simulink model "New_Control_Law_I_StandAlone"  (R2014a)
settings: configuration reference "AR_Drone_ConfigSet_NOEXT" (kept outside this file)
values from neighbouring files (symbols this model uses):
  Accel_Calib_Gain = Simulink.Parameter    [AR_DRONE_SCRIPT.m]
  Accel_Calib_Offset = Simulink.Parameter    [AR_DRONE_SCRIPT.m]
undefined symbols (not defined in the file or in its folder): Mag_Calib_Gain_Vector, Mag_Calib_Offset_Vector, Navigation, Navigation_KF_Lib, sigbuilder_block
libraries: simulink x14, vrlib x6, AR_Drone_2_Library x4, aerolibtransform2 x4, dspnetwork x4, aerolibutil x2
(part 1 of 3)
settings Model: ExtModeTrigDuration=48000  Creator=nraman  LastModifiedBy=darenlee

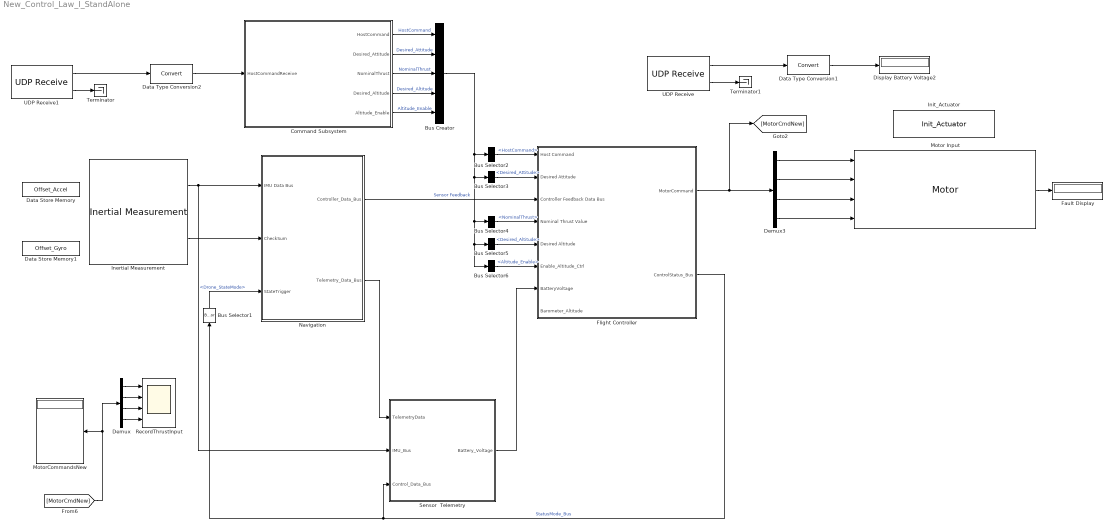
== system New_Control_Law_I_StandAlone ==
  Bus Creator : BusCreator  Inputs=5
  Bus Selector1 : BusSelector  OutputSignals=Drone_StateMode
  Bus Selector2 : BusSelector  OutputSignals=HostCommand
  Bus Selector3 : BusSelector  OutputSignals=Desired_Attitude
  Bus Selector4 : BusSelector  OutputSignals=NominalThrust
  Bus Selector5 : BusSelector  OutputSignals=Desired_Altitude
  Bus Selector6 : BusSelector  OutputSignals=Altitude_Enable
  Command Subsystem : Subsystem
  Data Store Memory : DataStoreMemory  DataStoreName=Offset_Accel  ReadBeforeWriteMsg=warning  WriteAfterWriteMsg=warning  WriteAfterReadMsg=warning  InitialValue=[0 0]  OutDataTypeStr=double
  Data Store Memory1 : DataStoreMemory  DataStoreName=Offset_Gyro  ReadBeforeWriteMsg=warning  WriteAfterWriteMsg=warning  WriteAfterReadMsg=warning  InitialValue=[0 0 0]  OutDataTypeStr=double
  Data Type Conversion1 : DataTypeConversion
  Data Type Conversion2 : DataTypeConversion
  Demux : Demux
  Demux3 : Demux
  Display Battery Voltage2 : Display
  Fault Display : Display
  Flight Controller : Subsystem
  Inertial Measurement : AR_Drone_2_Library/Inertial Measurement  Ts=1/400
  Init_Actuator : AR_Drone_2_Library/Init_Actuator  ShowSpec=on
  Motor Input : AR_Drone_2_Library/Motor
  MotorCommandsNew : Display
  Navigation : Subsystem  AncestorBlock=Navigation_KF_Lib/Navigation
      mask DialogControl DescTextVar Prompt: Kalman Filter Navigation Implementation
  RecordThrustInput : Scope  NumInputPorts=4
      settings: TimeRange=44.32823813354787  YMin=20~20~-5~-5  YMax=85~90~5~5  SaveName=Control_Input
  Sensor  Telemetry : Subsystem
  Terminator : Terminator
  Terminator1 : Terminator
  UDP Receive : dspnetwork/UDP Receive  localURL='0.0.0.0'  localPort=6000  remoteURL='192.168.1.2'  remotePort=-1  recvBufferSize=8192  dims=1  signalDatatype=int8  isVarSize=off  showBlockingTime=on  blockingTime=0  sampletime=1/400  blockPlatform=LINUX
  UDP Receive1 : dspnetwork/UDP Receive  localURL='0.0.0.0'  localPort=6000  remoteURL='192.168.1.2'  remotePort=-1  recvBufferSize=8192  dims=1  signalDatatype=int8  isVarSize=off  showBlockingTime=on  blockingTime=0  sampletime=1/400  blockPlatform=LINUX
  wires:
  Motor Input/1 -> Fault Display/1
  Demux3/1 -> Motor Input/1
  Demux3/2 -> Motor Input/2
  Demux3/3 -> Motor Input/3
  Demux3/4 -> Motor Input/4
  Inertial Measurement/1 -> Sensor  Telemetry/2(IMU_Bus), Navigation/1(IMU Data Bus)
  Inertial Measurement/2 -> Navigation/2(CheckSum)
  Bus Creator/1 -> Bus Selector2/1, Bus Selector3/1, Bus Selector4/1, Bus Selector6/1, Bus Selector5/1
  Bus Selector4/1 -> Flight Controller/4(Nominal Thrust Value)  "<NominalThrust>"
  Bus Selector5/1 -> Flight Controller/5(Desired Altitude)  "<Desired_Altitude>"
  Bus Selector6/1 -> Flight Controller/6(Enable_Altitude_Ctrl)  "<Altitude_Enable>"
  Flight Controller/1(MotorCommand) -> [MotorCmdNew], Demux3/1
  Flight Controller/2(ControlStatus_Bus) -> Sensor  Telemetry/3(Control_Data_Bus), Bus Selector1/1  "StatusMode_Bus"
  Bus Selector1/1 -> Navigation/3(StateTrigger)  "<Drone_StateMode>"
  [MotorCmdNew] -> MotorCommandsNew/1, Demux/1
  Demux/1 -> RecordThrustInput/1
  Demux/2 -> RecordThrustInput/2
  Demux/3 -> RecordThrustInput/3
  Demux/4 -> RecordThrustInput/4
  Command Subsystem/1(HostCommand) -> Bus Creator/1  "HostCommand"
  Command Subsystem/2(Desired_Attitude) -> Bus Creator/2  "Desired_Attitude"
  Command Subsystem/3(NominalThrust) -> Bus Creator/3  "NominalThrust"
  Command Subsystem/4(Desired_Altitude) -> Bus Creator/4  "Desired_Altitude"
  Command Subsystem/5(Altitude_Enable) -> Bus Creator/5  "Altitude_Enable"
  Bus Selector2/1 -> Flight Controller/1(Host Command)  "<HostCommand>"
  Bus Selector3/1 -> Flight Controller/2(Desired Attitude)  "<Desired_Attitude>"
  Navigation/1(Controller_Data_Bus) -> Flight Controller/3(Controller Feedback Data Bus)  "Sensor Feedback"
  Navigation/2(Telemetry_Data_Bus) -> Sensor  Telemetry/1(TelemetryData)
  UDP Receive/1 -> Data Type Conversion1/1
  Data Type Conversion1/1 -> Display Battery Voltage2/1
  Sensor  Telemetry/1(Battery_Voltage) -> Flight Controller/7(BatteryVoltage)
  UDP Receive1/1 -> Data Type Conversion2/1
  Data Type Conversion2/1 -> Command Subsystem/1(HostCommandReceive)
  UDP Receive1/2 -> Terminator/1
  UDP Receive/2 -> Terminator1/1

== system New_Control_Law_I_StandAlone/Command Subsystem ==
  HostCommandReceive : Inport
  Altitude_OFF : Constant  Value=0
  Altitude_ON : Constant
  Data Type Conversion5 : DataTypeConversion
  Desired Attitude : Subsystem
  Desired Euler Angle Attitude1 : Constant  Value=120
  Desired Euler Angle Attitude2 : Constant  Value=50
  Enable/Disable Altitude : ManualSwitch
  Go High : Constant
  Go Low : Constant  Value=0
  Height Control : ManualSwitch
  Nominal Thrust1 : Constant  Value=55
  Switch1 : Switch  Criteria=u2 > Threshold
  HostCommand : Outport
  Desired_Attitude : Outport  Port=2
  NominalThrust : Outport  Port=3
  Desired_Altitude : Outport  Port=4
  Altitude_Enable : Outport  Port=5
  wires:
  Desired Euler Angle Attitude2/1 -> Switch1/3
  Height Control/1 -> Switch1/2
  Desired Euler Angle Attitude1/1 -> Switch1/1
  Go High/1 -> Height Control/1
  Go Low/1 -> Height Control/2
  Altitude_OFF/1 -> Enable/Disable Altitude/2
  Altitude_ON/1 -> Enable/Disable Altitude/1
  Switch1/1 -> Desired_Altitude/1
  Enable/Disable Altitude/1 -> Altitude_Enable/1
  Nominal Thrust1/1 -> NominalThrust/1
  Desired Attitude/1(Ref_Attitude) -> Data Type Conversion5/1
  Data Type Conversion5/1 -> Desired_Attitude/1
  HostCommandReceive/1 -> HostCommand/1

== system New_Control_Law_I_StandAlone/Flight Controller ==
  Host Command : Inport
  Desired Attitude : Inport  Port=2
  Controller Feedback Data Bus : Inport  Port=3
  Nominal Thrust Value : Inport  Port=4
  Desired Altitude : Inport  Port=5
  Enable_Altitude_Ctrl : Inport  Port=6
  BatteryVoltage : Inport  Port=7
  Barometer_Altitude : Inport  Port=8
  Bus Creator : BusCreator  Inputs=5
  Bus Selector : BusSelector  OutputSignals=UltraSound,EulerAngles,ProcessedGyro,AccelNorm
  FilterBattVoltage : DiscreteTransferFcn  Numerator=[ 0.07226]  Denominator=[1 -0.9277]  SampleTime=1/400
  Selector : Selector  InputPortWidth=3  Indices=[3]
  Supervisory Flight Controller : Stateflow chart  TreatAsAtomicUnit=on
  Terminator : Terminator
  MotorCommand : Outport
  ControlStatus_Bus : Outport  Port=2
  wires:
  Supervisory Flight Controller/1(MotorCmd) -> Bus Creator/1, MotorCommand/1
  Desired Attitude/1 -> Supervisory Flight Controller/2(Desired_Attitude_deg)
  Desired Altitude/1 -> Supervisory Flight Controller/9(Desired_Altitude)
  Supervisory Flight Controller/2(" Drone_StateMode") -> Bus Creator/2
  Host Command/1 -> Supervisory Flight Controller/1(hostCmd)
  Bus Selector/1 -> Supervisory Flight Controller/3(UltraSound_Feedback)  "<UltraSound>"
  Nominal Thrust Value/1 -> Supervisory Flight Controller/7(NominalThrust)
  Controller Feedback Data Bus/1 -> Bus Selector/1
  Enable_Altitude_Ctrl/1 -> Supervisory Flight Controller/8(EnableAltitudeCtrl)
  [AccelOffset] -> Supervisory Flight Controller/11(Offset_Parameters)
  Supervisory Flight Controller/5(refHeight) -> Bus Creator/5
  [GyroOffset_Tag] -> Supervisory Flight Controller/12(GyroOffset_Parameters)
  BatteryVoltage/1 -> FilterBattVoltage/1
  FilterBattVoltage/1 -> Supervisory Flight Controller/10(Measured_Battery_Voltage)
  Selector/1 -> Supervisory Flight Controller/6(AccelVector_Input)
  Supervisory Flight Controller/3(" BatteryFault_Mode") -> Bus Creator/3
  Supervisory Flight Controller/4(" SafeOrientation_Mode") -> Bus Creator/4
  Bus Creator/1 -> ControlStatus_Bus/1  "StatusMode_Bus"
  Bus Selector/4 -> Selector/1  "<AccelNorm>"
  Bus Selector/2 -> Supervisory Flight Controller/4(Euler_Angles)  "<EulerAngles>"
  Bus Selector/3 -> Supervisory Flight Controller/5(Angular_Velocity)  "<ProcessedGyro>"
  Barometer_Altitude/1 -> Terminator/1

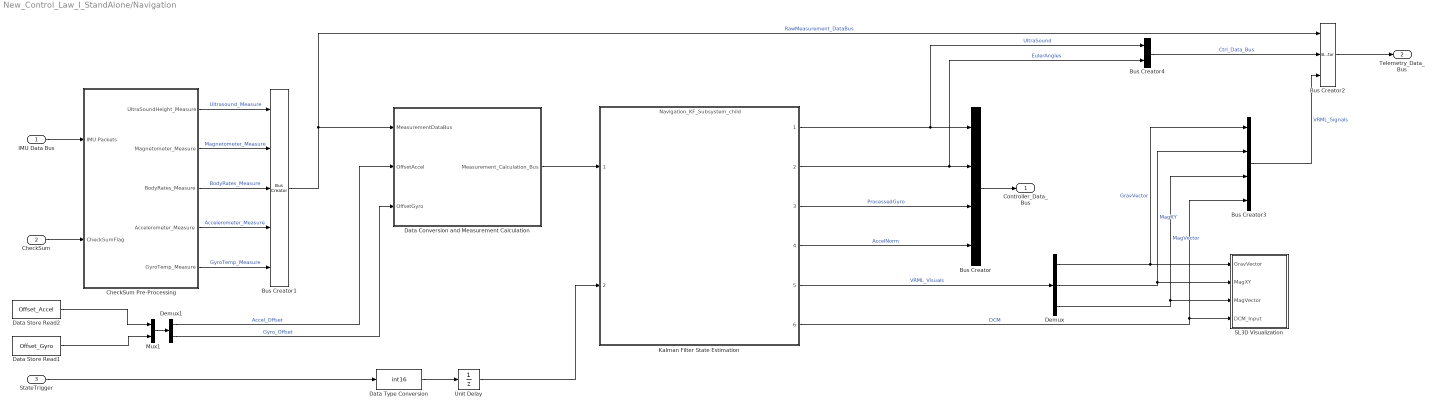
== system New_Control_Law_I_StandAlone/Navigation ==
  IMU Data Bus : Inport  OutDataTypeStr=Bus: IMU_Packets
  CheckSum : Inport  Port=2
  StateTrigger : Inport  Port=3  OutDataTypeStr=Enum: Drone_StateModeType
  Bus Creator : BusCreator
  Bus Creator1 : BusCreator  Inputs=5
  Bus Creator2 : BusCreator  Inputs=3
  Bus Creator3 : BusCreator
  Bus Creator4 : BusCreator  Inputs=2
  CheckSum Pre-Processing : Subsystem  TreatAsAtomicUnit=on
      settings: RTWSystemCode=Inline
  Data Conversion and Measurement Calculation : Subsystem
  Data Store Read1 : DataStoreRead  DataStoreName=Offset_Gyro
  Data Store Read2 : DataStoreRead  DataStoreName=Offset_Accel
  Data Type Conversion : DataTypeConversion  OutDataTypeStr=int16
  Demux : Demux  Outputs=[3 3 3]
  Demux1 : Demux  Outputs=[2 3]
  Kalman Filter State Estimation : ModelReference  ModelNameDialog=Navigation_KF_Subsystem_child.slx  SimulationMode=Normal  ModelReferenceVersion=1.55  CopyOfModelName=Navigation_KF_Subsystem_child.slx  DefaultDataLogging=on
  Mux1 : Mux  Inputs=2
  SL3D Visualization : Subsystem
  Unit Delay : UnitDelay  SampleTime=-1
  Controller_Data_Bus : Outport
  Telemetry_Data_Bus : Outport  Port=2
  wires:
  Kalman Filter State Estimation/4 -> Bus Creator/4  "AccelNorm"
  Kalman Filter State Estimation/3 -> Bus Creator/3  "ProcessedGyro"
  Data Conversion and Measurement Calculation/1(Measurement_Calculation_Bus) -> Kalman Filter State Estimation/1
  StateTrigger/1 -> Data Type Conversion/1
  Demux1/2 -> Data Conversion and Measurement Calculation/3(OffsetGyro)  "Gyro_Offset"
  Demux1/1 -> Data Conversion and Measurement Calculation/2(OffsetAccel)  "Accel_Offset"
  Mux1/1 -> Demux1/1
  Bus Creator1/1 -> Bus Creator2/1, Data Conversion and Measurement Calculation/1(MeasurementDataBus)  "RawMeasurement_DataBus"
  CheckSum Pre-Processing/5(GyroTemp_Measure) -> Bus Creator1/5  "GyroTemp_Measure"
  CheckSum Pre-Processing/4(Accelerometer_Measure) -> Bus Creator1/4  "Accelerometer_Measure"
  CheckSum Pre-Processing/3(BodyRates_Measure) -> Bus Creator1/3  "BodyRates_Measure"
  CheckSum Pre-Processing/2(Magnetometer_Measure) -> Bus Creator1/2  "Magnetometer_Measure"
  CheckSum Pre-Processing/1(UltraSoundHeight_Measure) -> Bus Creator1/1  "Ultrasound_Measure"
  CheckSum/1 -> CheckSum Pre-Processing/2(CheckSumFlag)
  IMU Data Bus/1 -> CheckSum Pre-Processing/1(IMU Packets)
  Unit Delay/1 -> Kalman Filter State Estimation/2
  Data Type Conversion/1 -> Unit Delay/1
  Kalman Filter State Estimation/6 -> Bus Creator3/4, SL3D Visualization/4(DCM_Input)  "DCM"
  Kalman Filter State Estimation/1 -> Bus Creator4/1, Bus Creator/1  "UltraSound"
  Demux/1 -> Bus Creator3/1, SL3D Visualization/1(GravVector)  "GravVector"
  Demux/3 -> Bus Creator3/3, SL3D Visualization/3(MagVector)  "MagVector"
  Bus Creator/1 -> Controller_Data_Bus/1
  Kalman Filter State Estimation/2 -> Bus Creator4/2, Bus Creator/2  "EulerAngles"
  Kalman Filter State Estimation/5 -> Demux/1  "VRML_Visuals"
  Data Store Read2/1 -> Mux1/1
  Data Store Read1/1 -> Mux1/2
  Bus Creator2/1 -> Telemetry_Data_Bus/1
  Bus Creator3/1 -> Bus Creator2/3  "VRML_Signals"
  Demux/2 -> Bus Creator3/2, SL3D Visualization/2(MagXY)  "MagXY"
  Bus Creator4/1 -> Bus Creator2/2  "Ctrl_Data_Bus"

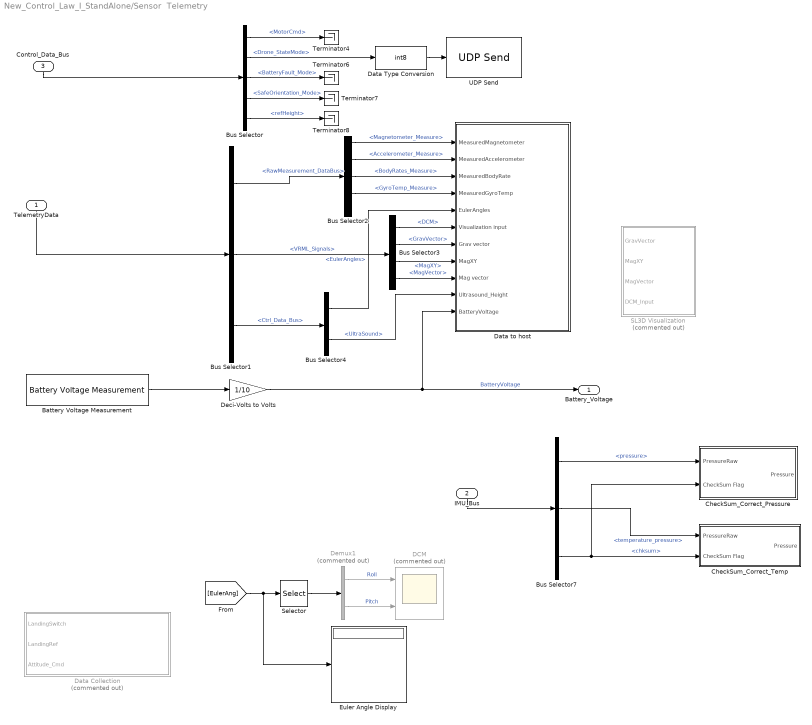
== system New_Control_Law_I_StandAlone/Sensor  Telemetry ==
  TelemetryData : Inport
  IMU_Bus : Inport  Port=2
  Control_Data_Bus : Inport  Port=3
  Battery Voltage Measurement : AR_Drone_2_Library/Battery Voltage Measurement  SFunctionSpec=void BatteryMeasure_step(single y1[1])  SampleTime=1/400
  Bus Selector : BusSelector  OutputSignals=MotorCmd,Drone_StateMode,BatteryFault_Mode,SafeOrientation_Mode,refHeight
  Bus Selector1 : BusSelector  OutputSignals=RawMeasurement_DataBus,VRML_Signals,Ctrl_Data_Bus
  Bus Selector2 : BusSelector  OutputSignals=Magnetometer_Measure,Accelerometer_Measure,BodyRates_Measure,GyroTemp_Measure,Ultrasound_Measure
  Bus Selector3 : BusSelector  OutputSignals=DCM,GravVector,MagXY,MagVector
  Bus Selector4 : BusSelector  OutputSignals=EulerAngles,UltraSound
  Bus Selector7 : BusSelector  OutputSignals=pressure,temperature_pressure,chksum
  CheckSum_Correct_Pressure : Subsystem
  CheckSum_Correct_Temp : Subsystem
  DCM : Scope  Commented=on  NumInputPorts=2
      settings: TimeRange=18.24617860016089  YMin=-20~-0.6  YMax=30~0.1  SaveName=EulerAngles
  Data Collection : Subsystem  Commented=on
  Data Type Conversion : DataTypeConversion  OutDataTypeStr=int8
  Data to host : Subsystem
  Deci-Volts to Volts : Gain  Gain=1/10
  Demux1 : Demux  Commented=on  Outputs=2
  Euler Angle Display : Display
  SL3D Visualization : Subsystem  Commented=on
  Selector : Selector  InputPortWidth=3  Indices=[1 2]
  Terminator{4,6..8} (4 alike) : Terminator
  UDP Send : dspnetwork/UDP Send  remoteURL='192.168.1.2'  remotePort=24000  localURL='0.0.0.0'  localPortSource=Automatically determine  localPort=-1  sampletime=-1  blockPlatform=LINUX  separateLengthPort=0
  Battery_Voltage : Outport
  wires:
  Battery Voltage Measurement/1 -> Deci-Volts to Volts/1
  Deci-Volts to Volts/1 -> Data to host/11(BatteryVoltage), Battery_Voltage/1  "BatteryVoltage"
  Bus Selector7/2 -> CheckSum_Correct_Temp/1(PressureRaw)  "<temperature_pressure>"
  IMU_Bus/1 -> Bus Selector7/1
  Bus Selector7/3 -> CheckSum_Correct_Pressure/2(CheckSum Flag), CheckSum_Correct_Temp/2(CheckSum Flag)  "<chksum>"
  Bus Selector7/1 -> CheckSum_Correct_Pressure/1(PressureRaw)  "<pressure>"
  Demux1/1 -> DCM/1  "Roll"
  Demux1/2 -> DCM/2  "Pitch"
  [EulerAng] -> Selector/1, Euler Angle Display/1
  Selector/1 -> Demux1/1
  TelemetryData/1 -> Bus Selector1/1
  Bus Selector/1 -> Terminator4/1  "<MotorCmd>"
  Bus Selector/3 -> Terminator6/1  "<BatteryFault_Mode>"
  Bus Selector/4 -> Terminator7/1  "<SafeOrientation_Mode>"
  Bus Selector/5 -> Terminator8/1  "<refHeight>"
  Bus Selector1/1 -> Bus Selector2/1  "<RawMeasurement_DataBus>"
  Bus Selector1/2 -> Bus Selector3/1  "<VRML_Signals>"
  Bus Selector3/1 -> Data to host/6(Visualization input)  "<DCM>"
  Bus Selector3/2 -> Data to host/7(Grav vector)  "<GravVector>"
  Bus Selector3/3 -> Data to host/8(MagXY)  "<MagXY>"
  Bus Selector3/4 -> Data to host/9(Mag vector)  "<MagVector>"
  Bus Selector2/1 -> Data to host/1(MeasuredMagnetometer)  "<Magnetometer_Measure>"
  Bus Selector2/2 -> Data to host/2(MeasuredAccelerometer)  "<Accelerometer_Measure>"
  Bus Selector2/3 -> Data to host/3(MeasuredBodyRate)  "<BodyRates_Measure>"
  Bus Selector2/4 -> Data to host/4(MeasuredGyroTemp)  "<GyroTemp_Measure>"
  Bus Selector1/3 -> Bus Selector4/1  "<Ctrl_Data_Bus>"
  Bus Selector4/1 -> Data to host/5(EulerAngles)  "<EulerAngles>"
  Bus Selector4/2 -> Data to host/10(Ultrasound_Height)  "<UltraSound>"
  Data Type Conversion/1 -> UDP Send/1
  Control_Data_Bus/1 -> Bus Selector/1
  Bus Selector/2 -> Data Type Conversion/1  "<Drone_StateMode>"

== system New_Control_Law_I_StandAlone/Command Subsystem/Desired Attitude ==
  Desired Euler Angle Attitude : Constant  Value=0
  Mux2 : Mux  Inputs=3
  Ref_Attitude : Outport
  wires:
  Desired Euler Angle Attitude/1 -> Mux2/3, Mux2/2, Mux2/1
  Mux2/1 -> Ref_Attitude/1

== system New_Control_Law_I_StandAlone/Flight Controller/Supervisory Flight Controller/Altitude_Control ==
  note: Thurst Table
      | _________________
      | At 100cm error  - 20% duty cycle - saturation : 10
      | 80 cm error - 16% duty cycle - saturation
      | 70 cm error - 14% duty cycle - saturation
      | 60 cm error - 12% duty cycle
  HeightFeedback : Inport  OutDataTypeStr=double  PortDimensions=2
  refHeight : Inport  Port=2  OutDataTypeStr=double  PortDimensions=1
  f : TriggerPort  TriggerType=function-call
      settings: CopyFcn=Stateflow.SLINSF.SimulinkMan.removeBlockPreDeleteFcn  PreDeleteFcn=Stateflow.SLINSF.SimulinkMan.unsafePredeleteFcn
  Control Effort : Scope
      settings: YMin=8.735  YMax=8.7875  SaveName=ScopeData3
  Data Type Conversion1 : DataTypeConversion  OutDataTypeStr=int16
  Demux : Demux  Outputs=2
  Discrete PID Controller _ WORKING1 : simulink/Continuous/PID Controller  Commented=on  Controller=PID  TimeDomain=Discrete-time  SampleTime=-1  IntegratorMethod=Forward Euler  FilterMethod=Forward Euler  Form=Parallel  P=0.387369235850492*0.7  I=0.018136*4  D=0.819231727791919*0.15  N=12.5907330811849  InitialConditionSource=internal  InitialConditionForIntegrator=0  InitialConditionForFilter=0  ExternalReset=none  LimitOutput=on  UpperSaturationLimit=20  LowerSaturationLimit=-20  LinearizeAsGain=off  AntiWindupMode=clamping  Kb=1  TrackingMode=off  Kt=1  PParamMin=[]  PParamMax=[]  IParamMin=[]  IParamMax=[]  DParamMin=[]  DParamMax=[]  NParamMin=[]  NParamMax=[]  KbParamMin=[]  KbParamMax=[]  KtParamMin=[]  KtParamMax=[]  POutMin=[]  POutMax=[]  IOutMin=[]  IOutMax=[]  DOutMin=[]  DOutMax=[]  NOutMin=[]  NOutMax=[]  KbOutMin=[]  KbOutMax=[]  KtOutMin=[]  KtOutMax=[]  IntegratorOutMin=[]  IntegratorOutMax=[]  FilterOutMin=[]  FilterOutMax=[]  SumOutMin=[]  SumOutMax=[]  SumI1OutMin=[]  SumI1OutMax=[]  SumI2OutMin=[]  SumI2OutMax=[]  SumI3OutMin=[]  SumI3OutMax=[]  SumDOutMin=[]  SumDOutMax=[]  SaturationOutMin=[]  SaturationOutMax=[]  IntegratorContinuousStateAttributes=''  IntegratorStateMustResolveToSignalObject=off  IntegratorRTWStateStorageClass=Auto  FilterContinuousStateAttributes=''  FilterStateMustResolveToSignalObject=off  FilterRTWStateStorageClass=Auto
  Display3 : Display
  Height Error : Scope  NumInputPorts=2
      settings: ShowLegends=on  YMin=-0.1075~-5  YMax=-0.08~5  SaveName=ScopeData13
  PID_Smooth : simulink/Continuous/PID Controller  Controller=PID  TimeDomain=Discrete-time  SampleTime=-1  IntegratorMethod=Forward Euler  FilterMethod=Forward Euler  Form=Parallel  P=0.387369235850492*0.9  I=0.018136*4  D=0.819231727791919*0.2  N=12.5907330811849  InitialConditionSource=internal  InitialConditionForIntegrator=0  InitialConditionForFilter=0  ExternalReset=none  LimitOutput=on  UpperSaturationLimit=20  LowerSaturationLimit=-20  LinearizeAsGain=off  AntiWindupMode=clamping  Kb=1  TrackingMode=off  Kt=1  PParamMin=[]  PParamMax=[]  IParamMin=[]  IParamMax=[]  DParamMin=[]  DParamMax=[]  NParamMin=[]  NParamMax=[]  KbParamMin=[]  KbParamMax=[]  KtParamMin=[]  KtParamMax=[]  POutMin=[]  POutMax=[]  IOutMin=[]  IOutMax=[]  DOutMin=[]  DOutMax=[]  NOutMin=[]  NOutMax=[]  KbOutMin=[]  KbOutMax=[]  KtOutMin=[]  KtOutMax=[]  IntegratorOutMin=[]  IntegratorOutMax=[]  FilterOutMin=[]  FilterOutMax=[]  SumOutMin=[]  SumOutMax=[]  SumI1OutMin=[]  SumI1OutMax=[]  SumI2OutMin=[]  SumI2OutMax=[]  SumI3OutMin=[]  SumI3OutMax=[]  SumDOutMin=[]  SumDOutMax=[]  SaturationOutMin=[]  SaturationOutMax=[]  IntegratorContinuousStateAttributes=''  IntegratorStateMustResolveToSignalObject=off  IntegratorRTWStateStorageClass=Auto  FilterContinuousStateAttributes=''  FilterStateMustResolveToSignalObject=off  FilterRTWStateStorageClass=Auto
  Re-Calibrate : Saturate  UpperLimit=200  LowerLimit=0  OutMin=0  OutMax=200
      settings: AttributesFormatString=|
      | Upper: %<UpperLimit>
      | Lower %<LowerLimit>
  Sum : Sum  Inputs=|-+
  deltaThrottle : Outport  OutDataTypeStr=int16
  wires:
  refHeight/1 -> Sum/2, Height Error/2, Display3/1  "Commanded"
  PID_Smooth/1 -> Control Effort/1, Data Type Conversion1/1
  Data Type Conversion1/1 -> deltaThrottle/1
  HeightFeedback/1 -> Demux/1
  Demux/1 -> Re-Calibrate/1
  Sum/1 -> PID_Smooth/1, Height Error/1  "Error"
  Re-Calibrate/1 -> Sum/1

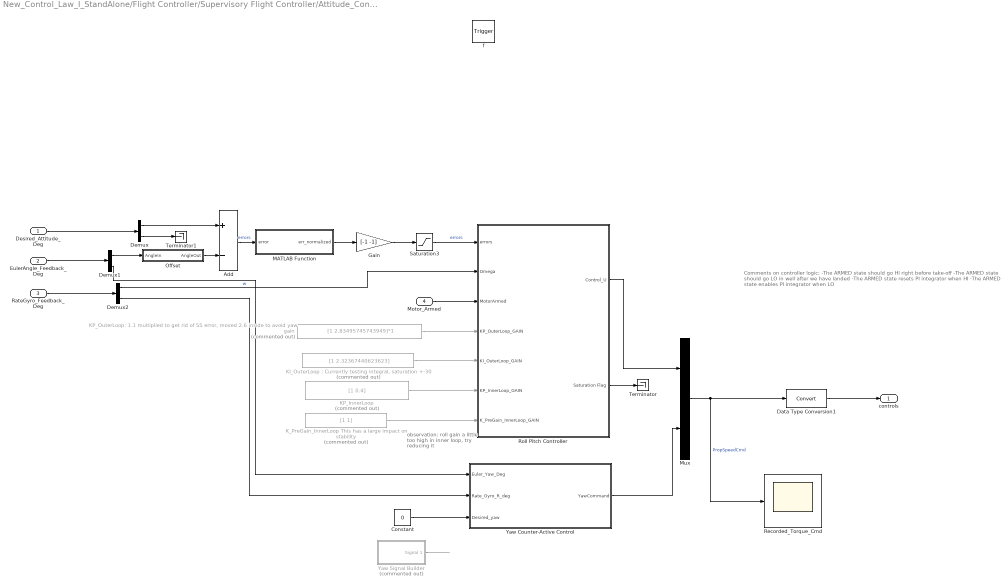
== system New_Control_Law_I_StandAlone/Flight Controller/Supervisory Flight Controller/Attitude_Control ==
  note: observation:
      | roll gain a little
      | too high in inner
      | loop, try reducing it
  note: Comments on controller logic:
      | -The ARMED state should go HI right before take-off
      | -The  ARMED state should go LO in well after we have landed
      | -The ARMED state resets PI integrator when HI
      | -The ARMED state enables PI integrator when LO
  Desired_Attitude_Deg : Inport  OutDataTypeStr=double  PortDimensions=3
  EulerAngle_Feedback_Deg : Inport  Port=2  OutDataTypeStr=double  PortDimensions=3
  RateGyro_Feedback_Deg : Inport  Port=3  OutDataTypeStr=double  PortDimensions=3
  Motor_Armed : Inport  Port=4  OutDataTypeStr=double  PortDimensions=1
  f : TriggerPort  TriggerType=function-call
      settings: CopyFcn=Stateflow.SLINSF.SimulinkMan.removeBlockPreDeleteFcn  PreDeleteFcn=Stateflow.SLINSF.SimulinkMan.unsafePredeleteFcn
  Add : Sum  Inputs=+-  AccumDataTypeStr=single  OutDataTypeStr=single
  Constant : Constant  Value=0
  Data Type Conversion1 : DataTypeConversion
  Demux : Demux  Outputs=[2 1]
  Demux1 : Demux  Outputs=[2 1]
  Demux2 : Demux  Outputs=[2 1]
  Gain : Gain  Gain=[-1 -1]
  "KI_OuterLoop : Currently testing integral, saturation +-30" : Constant  Commented=on  Value=[1 2.32367440623623]
  KP_InnerLoop : Constant  Commented=on  Value=[1 0.4]
  "KP_OuterLoop: 1.1 multiplied to get rid of SS error, moved 2.6 inside to avoid yaw gain" : Constant  Commented=on  Value=[1 2.83495745743949]*1
  K_PreGain_InnerLoop This has a large impact on stability : Constant  Commented=on  Value=[1 1]
  MATLAB Function : MATLAB Function  TreatAsAtomicUnit=on
  Mux : Mux  Inputs=2
  Offset : Subsystem
  Recorded_Torque_Cmd : Scope
      settings: TimeRange=30  YMin=-30  YMax=30  SaveName=Toqrue_Input
  Roll Pitch Controller : Subsystem  TreatAsAtomicUnit=on
  Saturation3 : Saturate  UpperLimit=[25 25]  LowerLimit=[-25 -25]  OutDataTypeStr=single
      settings: AttributesFormatString=%<LowerLimit> to %<UpperLimit>
  Terminator : Terminator
  Terminator1 : Terminator
  Yaw Counter-Active Control : Subsystem
  "Yaw Signal Builder " : Subsystem  Tag=STV Subsys  Commented=on  LoadFcn=sigbuilder_block('load');  StartFcn=sigbuilder_block('start');  StopFcn=sigbuilder_block('stop');  ClipboardFcn=sigbuilder_block('clipboard');  mask(Sigbuilder block){}
      mask help: Simulink:masks:SigbuilderBlock_MD
      mask init:
      | if ~strcmp(get_param(bdroot(gcbh),'SimulationStatus'),'stopped') tuvar = sigbuilder_block('maskInit'); end
      settings: CopyFcn=sigbuilder_block('copy');  DeleteFcn=sigbuilder_block('delete');  ModelCloseFcn=sigbuilder_block('modelClose');  PreSaveFcn=sigbuilder_block('preSave');  PauseFcn=sigbuilder_block('pause');  ContinueFcn=sigbuilder_block('continue');  NameChangeFcn=sigbuilder_block('namechange');  OpenFcn=sigbuilder_block('open',[437.25 118.5 550.5 394.5 ]);  CloseFcn=sigbuilder_block('close');
      mask Display: plot(0, 0, 100, 100,[2, 2, 32, 32, 2], [68, 8, 8, 68, 68],[32, 2], [38, 38], [32, 19, 2],[53, 60, 44], [32, 17, 17, 2],[16, 16, 31, 31]);txt = getActiveGroup(gcbh);text(2, 100, txt,'verticalAlignment', 'top');
  controls : Outport  OutDataTypeStr=int16  PortDimensions=3  InitialOutput=0
  wires:
  Add/1 -> MATLAB Function/1(error)  "errors"
  Demux1/1 -> Offset/1(AngleIn)
  Demux2/1 -> Roll Pitch Controller/2(Omega)  "w"
  KP_InnerLoop/1 -> Roll Pitch Controller/6(KP_InnerLoop_GAIN)
  "KP_OuterLoop: 1.1 multiplied to get rid of SS error, moved 2.6 inside to avoid yaw gain"/1 -> Roll Pitch Controller/4(KP_OuterLoop_GAIN)
  K_PreGain_InnerLoop This has a large impact on stability/1 -> Roll Pitch Controller/7(K_PreGain_InnerLoop_GAIN)
  "KI_OuterLoop : Currently testing integral, saturation +-30"/1 -> Roll Pitch Controller/5(KI_OuterLoop_GAIN)
  Saturation3/1 -> Roll Pitch Controller/1(errors)  "errors"
  MATLAB Function/1(err_normalized) -> Gain/1
  Gain/1 -> Saturation3/1
  Roll Pitch Controller/2(Saturation Flag) -> Terminator/1
  Demux/1 -> Add/1
  Roll Pitch Controller/1(Control_U) -> Mux/1
  Demux/2 -> Terminator1/1
  Offset/1(AngleOut) -> Add/2
  Demux2/2 -> Yaw Counter-Active Control/2(Rate_Gyro_R_deg)
  Yaw Counter-Active Control/1(YawCommand) -> Mux/2
  Desired_Attitude_Deg/1 -> Demux/1
  EulerAngle_Feedback_Deg/1 -> Demux1/1
  RateGyro_Feedback_Deg/1 -> Demux2/1
  Motor_Armed/1 -> Roll Pitch Controller/3(MotorArmed)
  Demux1/2 -> Yaw Counter-Active Control/1(Euler_Yaw_Deg)
  Data Type Conversion1/1 -> controls/1
  Mux/1 -> Data Type Conversion1/1, Recorded_Torque_Cmd/1  "PropSpeedCmd"
  "Yaw Signal Builder "/1(Signal 1) -> ?
  Constant/1 -> Yaw Counter-Active Control/3("Desired_yaw ")

== system New_Control_Law_I_StandAlone/Flight Controller/Supervisory Flight Controller/Drone_State.Initialize.checkConvergence ==
  Euler_Angles : Inport  OutDataTypeStr=double  PortDimensions=3
  f : TriggerPort  TriggerType=function-call
      settings: CopyFcn=Stateflow.SLINSF.SimulinkMan.removeBlockPreDeleteFcn  PreDeleteFcn=Stateflow.SLINSF.SimulinkMan.unsafePredeleteFcn
  Compare To Constant : simulink/Logic and Bit Operations/Compare To Constant  relop=<  const=0.00001  OutDataTypeStr=boolean
  Delay : Delay  DelayLength=1  InitialCondition=inf
  Demux : Demux  Outputs=3
  Display : Display
  Logical Operator : Logic  Inputs=3  AllPortsSameDT=off  OutDataTypeStr=boolean
  Sum : Sum  Inputs=|+-
  dt : Gain  Gain=1/400
  converge : Outport
  wires:
  Euler_Angles/1 -> Sum/2, Delay/1
  Delay/1 -> Sum/1
  Sum/1 -> dt/1
  dt/1 -> Compare To Constant/1
  Compare To Constant/1 -> Display/1, Demux/1
  Logical Operator/1 -> converge/1
  Demux/1 -> Logical Operator/1
  Demux/2 -> Logical Operator/2
  Demux/3 -> Logical Operator/3

== system New_Control_Law_I_StandAlone/Flight Controller/Supervisory Flight Controller/Motor_Mixing ==
  note: AR Drone:
      |
      |   1x         2y
      |      drone
      |   4y         3x
      |
      |  1 = constrain(throttle + 0.5*roll - 0.5*pitch - yaw , minThrottle, 30);
      |  2 = constrain(throttle - 0.5*roll - 0.5*pitch + yaw, minThrottle, 30);
      |  3 = constrain(throttle - 0.5*roll + 0.5*pitch - yaw, minThrottle, 30);
      |  4 = constrain(throttle + 0.5*roll + 0.5*pitch + yaw, minThrottle, 30);
  throttle : Inport  OutDataTypeStr=int16  PortDimensions=1
  RPYCmd : Inport  Port=2  OutDataTypeStr=int16  PortDimensions=3
  LandingPhase : Inport  Port=3  OutDataTypeStr=double  PortDimensions=1
  Motor_Armed : Inport  Port=4  OutDataTypeStr=double  PortDimensions=1
  f : TriggerPort  TriggerType=function-call
      settings: CopyFcn=Stateflow.SLINSF.SimulinkMan.removeBlockPreDeleteFcn  PreDeleteFcn=Stateflow.SLINSF.SimulinkMan.unsafePredeleteFcn
  Constant : Constant  Value=100  OutDataTypeStr=int16  SampleTime=-1
  Constant1 : Constant  Value=[0 0 0 0]  OutDataTypeStr=int16
  Constant2 : Constant  Value=[55 55 55 55]*0.4
  Data Type Conversion : DataTypeConversion  OutDataTypeStr=double
  Gain : Gain  Gain=[1 1 -1 -1; 1 -1 -1 1; 1 -1 1 -1; 1 1 1 1]  Multiplication=Matrix(K*u)  ParamDataTypeStr=int16  OutDataTypeStr=int16
  Logical Operator1 : Logic  Operator=NOT  AllPortsSameDT=off  OutDataTypeStr=boolean
  Mux1 : Mux  Inputs=2
  RampDownInSpeed1 : MATLAB Function  TreatAsAtomicUnit=on
  Saturation Dynamic : simulink/Discontinuities/Saturation Dynamic  OutMin=[]  OutMax=[]  OutDataTypeStr=Inherit: Same as second input  OutDataType=fixdt(1, 16)  OutScaling=2^-10  DoSatur=off
  Switch : Switch  Criteria=u2 > Threshold
  Switch1 : Switch  Criteria=u2 > Threshold
  minThrottle : Constant  Value=10  OutDataTypeStr=int16
  MotorCommands : Outport  InitialOutput=0
  wires:
  RPYCmd/1 -> Mux1/2
  minThrottle/1 -> Saturation Dynamic/3
  Constant/1 -> Saturation Dynamic/1
  Mux1/1 -> Gain/1
  Gain/1 -> Saturation Dynamic/2
  throttle/1 -> Mux1/1
  Data Type Conversion/1 -> RampDownInSpeed1/1(Cmd)
  RampDownInSpeed1/1(motorCmd) -> Switch/3
  Constant2/1 -> Data Type Conversion/1
  LandingPhase/1 -> RampDownInSpeed1/2(stopCmd), Logical Operator1/1  "if 1==Land, if 0 == dont land"
  Switch/1 -> MotorCommands/1
  Logical Operator1/1 -> Switch/2
  Saturation Dynamic/1 -> Switch1/1
  Motor_Armed/1 -> Switch1/2
  Constant1/1 -> Switch1/3
  Switch1/1 -> Switch/1

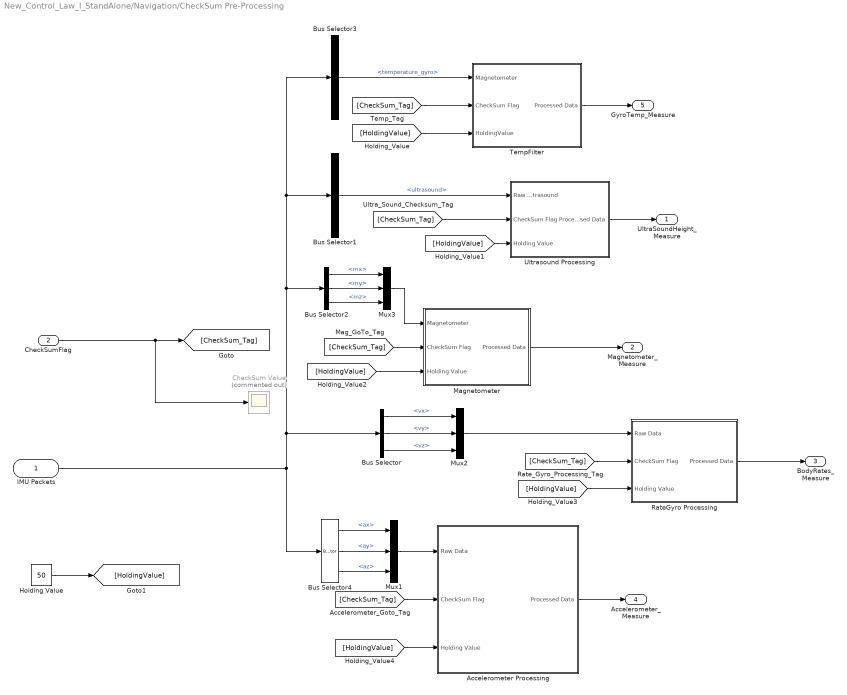
== system New_Control_Law_I_StandAlone/Navigation/CheckSum Pre-Processing ==
  IMU Packets : Inport
  CheckSumFlag : Inport  Port=2
  Accelerometer Processing : Subsystem
  Bus Selector : BusSelector  OutputSignals=vx,vy,vz
  Bus Selector1 : BusSelector  OutputSignals=ultrasound
  Bus Selector2 : BusSelector  OutputSignals=mx,my,mz
  Bus Selector3 : BusSelector  OutputSignals=temperature_gyro
  Bus Selector4 : BusSelector  OutputSignals=ax,ay,az
  CheckSum Value : Scope  Commented=on
      settings: YMin=0  YMax=2500  SaveName=CheckSum
  Holding Value : Constant  Value=50
  Magnetometer : Subsystem
  Mux1 : Mux  Inputs=3
  Mux2 : Mux  Inputs=3
  Mux3 : Mux  Inputs=3
  RateGyro Processing : Subsystem
  TempFilter : Subsystem
  Ultrasound Processing : Subsystem
  UltraSoundHeight_Measure : Outport
  Magnetometer_Measure : Outport  Port=2
  BodyRates_Measure : Outport  Port=3
  Accelerometer_Measure : Outport  Port=4
  GyroTemp_Measure : Outport  Port=5
  wires:
  Mux3/1 -> Magnetometer/1(Magnetometer)
  Holding Value/1 -> [HoldingValue]
  [HoldingValue] -> Accelerometer Processing/3(Holding Value)
  [HoldingValue] -> RateGyro Processing/3(Holding Value)
  [HoldingValue] -> Magnetometer/3(Holding Value)
  [HoldingValue] -> Ultrasound Processing/3(Holding Value)
  [HoldingValue] -> TempFilter/3(HoldingValue)
  [CheckSum_Tag] -> TempFilter/2(CheckSum Flag)
  TempFilter/1(Processed Data) -> GyroTemp_Measure/1
  Bus Selector3/1 -> TempFilter/1(Magnetometer)  "<temperature_gyro>"
  Bus Selector/3 -> Mux2/3  "<vz>"
  Bus Selector/2 -> Mux2/2  "<vy>"
  Bus Selector/1 -> Mux2/1  "<vx>"
  Ultrasound Processing/1(Processed Data) -> UltraSoundHeight_Measure/1
  [CheckSum_Tag] -> Accelerometer Processing/2(CheckSum Flag)
  Magnetometer/1(Processed Data) -> Magnetometer_Measure/1
  [CheckSum_Tag] -> Magnetometer/2(CheckSum Flag)
  Bus Selector2/3 -> Mux3/3  "<mz>"
  Bus Selector2/2 -> Mux3/2  "<my>"
  Bus Selector2/1 -> Mux3/1  "<mx>"
  RateGyro Processing/1(Processed Data) -> BodyRates_Measure/1
  [CheckSum_Tag] -> RateGyro Processing/2(CheckSum Flag)
  Mux2/1 -> RateGyro Processing/1(Raw Data)
  Accelerometer Processing/1(Processed Data) -> Accelerometer_Measure/1
  [CheckSum_Tag] -> Ultrasound Processing/2(CheckSum Flag)
  Mux1/1 -> Accelerometer Processing/1(Raw Data)
  Bus Selector4/3 -> Mux1/3  "<az>"
  Bus Selector4/2 -> Mux1/2  "<ay>"
  Bus Selector4/1 -> Mux1/1  "<ax>"
  IMU Packets/1 -> Bus Selector4/1, Bus Selector2/1, Bus Selector1/1, Bus Selector3/1, Bus Selector/1
  CheckSumFlag/1 -> CheckSum Value/1, [CheckSum_Tag]
  Bus Selector1/1 -> Ultrasound Processing/1(Raw Ultrasound)  "<ultrasound>"

== system New_Control_Law_I_StandAlone/Navigation/Data Conversion and Measurement Calculation ==
  MeasurementDataBus : Inport
  OffsetAccel : Inport  Port=2
  OffsetGyro : Inport  Port=3
  Bus Creator1 : BusCreator
  Bus Selector : BusSelector  OutputSignals=Ultrasound_Measure,Accelerometer_Measure,BodyRates_Measure,Magnetometer_Measure
  Calculate Gravity Vector : Subsystem
  Calibration_Scale_and_Offset : Subsystem
  Remove Offset : Subsystem
  Signal Specification : SignalSpecification
  Measurement_Calculation_Bus : Outport
  wires:
  MeasurementDataBus/1 -> Bus Selector/1
  Bus Selector/4 -> Calibration_Scale_and_Offset/1(RawMag)  "<Magnetometer_Measure>"
  OffsetAccel/1 -> Calculate Gravity Vector/2(Accel_Offset)
  OffsetGyro/1 -> Remove Offset/2(Gyro Offset)
  Bus Selector/3 -> Remove Offset/1(Raw Gyro Values)  "<BodyRates_Measure>"
  Bus Selector/1 -> Signal Specification/1  "<Ultrasound_Measure>"
  Calibration_Scale_and_Offset/1(Normalized  Magnetometer) -> Bus Creator1/4  "Magnetometer_Calculation"
  Remove Offset/1(Gyro Offset Remove) -> Bus Creator1/3  "Gyro_Calculation"
  Signal Specification/1 -> Bus Creator1/1  "UltraSound_Calculation"
  Calculate Gravity Vector/1(Accel_Norm) -> Bus Creator1/2  "AccelNorm_Calculation"
  Bus Creator1/1 -> Measurement_Calculation_Bus/1
  Bus Selector/2 -> Calculate Gravity Vector/1(Accel)  "<Accelerometer_Measure>"

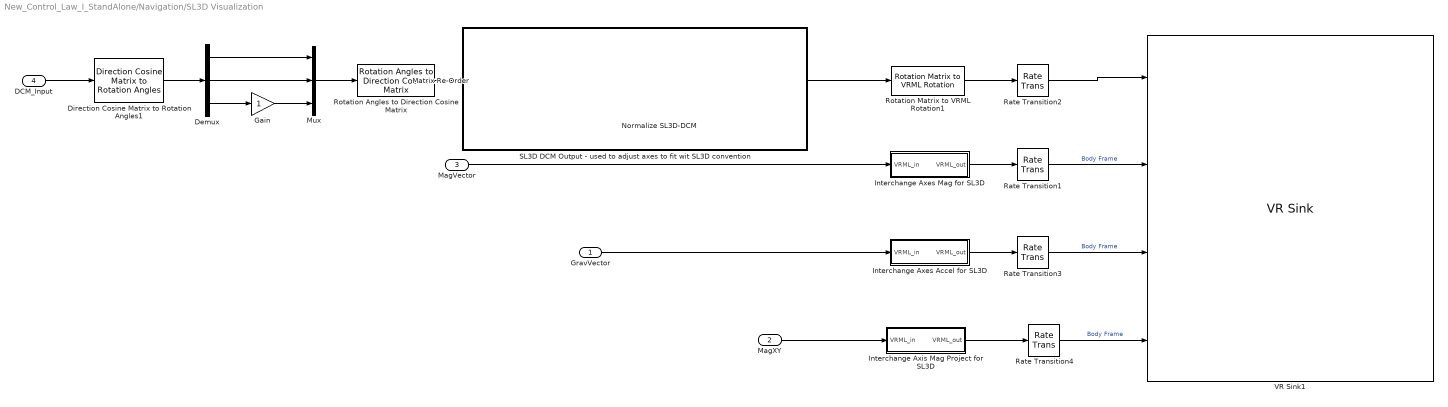
== system New_Control_Law_I_StandAlone/Navigation/SL3D Visualization ==
  GravVector : Inport
  MagXY : Inport  Port=2
  MagVector : Inport  Port=3
  DCM_Input : Inport  Port=4
  Demux : Demux  Outputs=3
  Direction Cosine Matrix to Rotation Angles1 : aerolibtransform2/Direction Cosine Matrix to Rotation Angles  rotationOrder=XYZ  lim=ZeroR3
      settings: AttributesFormatString=Rotation Order: %<rotationOrder>
  Gain : Gain  OutDataTypeStr=Inherit: Same as input
  "Interchange Axes Accel for SL3D " : Subsystem
  "Interchange Axes Mag for SL3D " : Subsystem
  Interchange Axis Mag Project for SL3D : Subsystem
  Matrix Re-Order : MATLAB Function  TreatAsAtomicUnit=on
  Mux : Mux  Inputs=3
  Normalize SL3D-DCM : Subsystem  TreatAsAtomicUnit=on
  Rate Transition{1..4} (4 alike) : RateTransition
  Rotation Angles to Direction Cosine Matrix : aerolibtransform2/Rotation Angles to Direction Cosine Matrix  rotationOrder=XYZ
  Rotation Matrix to VRML Rotation1 : vrlib/Utilities/Rotation Matrix to VRML Rotation  maxzero=1e-12
  SL3D DCM Output - used to adjust axes to fit wit SL3D convention : Subsystem
  VR Sink1 : vrlib/VR Sink  InstantiateOnLoad=on  SampleTime=0.02  ViewEnable=on  RemoteChange=off  RemoteView=off  FieldsWritten=Plane.rotation.4.1.1.double#mag_point.translation.3.1.1.double#grav_point.translation.3.1.1.double#mag_projection_point.translation.3.1.1.double  WorldFileName=vrml8_grav_2.WRL  AutoView=off  VideoDimensions=[]  AllowVariableSize=off
  wires:
  MagXY/1 -> Interchange Axis Mag Project for SL3D/1(VRML_in)
  Rate Transition2/1 -> VR Sink1/1
  Rate Transition1/1 -> VR Sink1/2  "Body Frame"
  Rate Transition3/1 -> VR Sink1/3  "Body Frame"
  Rate Transition4/1 -> VR Sink1/4  "Body Frame"
  Interchange Axis Mag Project for SL3D/1(VRML_out) -> Rate Transition4/1
  Rotation Angles to Direction Cosine Matrix/1 -> Matrix Re-Order/1(M_in)
  MagVector/1 -> "Interchange Axes Mag for SL3D "/1(VRML_in)
  "Interchange Axes Mag for SL3D "/1(VRML_out) -> Rate Transition1/1
  Mux/1 -> Rotation Angles to Direction Cosine Matrix/1
  Gain/1 -> Mux/3
  Demux/3 -> Gain/1
  Demux/2 -> Mux/2
  Demux/1 -> Mux/1
  Direction Cosine Matrix to Rotation Angles1/1 -> Demux/1
  Normalize SL3D-DCM/1(DCM_normalized) -> Rotation Matrix to VRML Rotation1/1
  Matrix Re-Order/1(M_out) -> Normalize SL3D-DCM/1(DCM)
  GravVector/1 -> "Interchange Axes Accel for SL3D "/1(VRML_in)
  DCM_Input/1 -> Direction Cosine Matrix to Rotation Angles1/1
  "Interchange Axes Accel for SL3D "/1(VRML_out) -> Rate Transition3/1
  Rotation Matrix to VRML Rotation1/1 -> Rate Transition2/1

== system New_Control_Law_I_StandAlone/Sensor  Telemetry/CheckSum_Correct_Pressure ==
  PressureRaw : Inport
  CheckSum Flag : Inport  Port=2
  CheckSum Correction : Subsystem
  Constant : Constant  Value=50
  Pressure : Outport
  wires:
  CheckSum Flag/1 -> CheckSum Correction/2(CheckSumFlag)
  CheckSum Correction/1(Pre-Processed Height) -> Pressure/1
  Constant/1 -> CheckSum Correction/3(Holding Value)
  PressureRaw/1 -> CheckSum Correction/1(CalculatedData)

== system New_Control_Law_I_StandAlone/Sensor  Telemetry/CheckSum_Correct_Temp ==
  PressureRaw : Inport
  CheckSum Flag : Inport  Port=2
  CheckSum Correction : Subsystem
  Constant : Constant  Value=50
  Pressure : Outport
  wires:
  CheckSum Flag/1 -> CheckSum Correction/2(CheckSumFlag)
  CheckSum Correction/1(Pre-Processed Height) -> Pressure/1
  Constant/1 -> CheckSum Correction/3(Holding Value)
  PressureRaw/1 -> CheckSum Correction/1(CalculatedData)

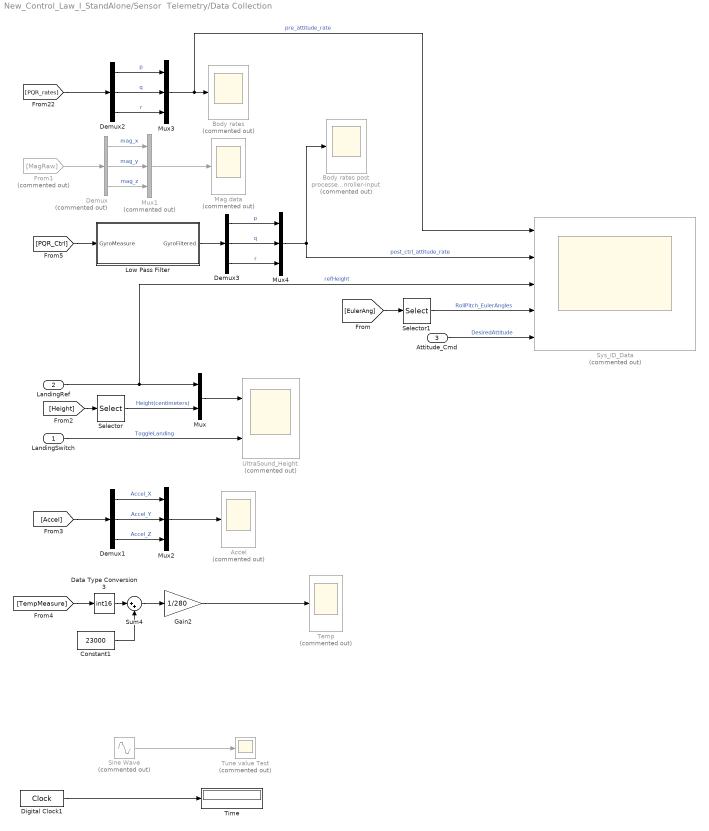
== system New_Control_Law_I_StandAlone/Sensor  Telemetry/Data Collection ==
  LandingSwitch : Inport
  LandingRef : Inport  Port=2
  Attitude_Cmd : Inport  Port=3
  Accel : Scope  Commented=on
      settings: ShowLegends=on  TimeRange=100  YMin=1850  YMax=2750  SaveName=Accel
  Body rates : Scope  Commented=on
      settings: ShowLegends=on  TimeRange=90  YMin=-1000  YMax=1200  SaveName=Gyro
  Body rates post processed - pre-conroller-input : Scope  Commented=on
      settings: ShowLegends=on  TimeRange=90  YMin=-1000  YMax=1200  SaveName=Gyro_PostProcessed
  Constant1 : Constant  Value=23000  OutDataTypeStr=int16
  Data Type Conversion3 : DataTypeConversion  OutDataTypeStr=int16
  Demux : Demux  Commented=on  Outputs=3
  Demux1 : Demux  Outputs=3
  Demux2 : Demux  Outputs=3
  Demux3 : Demux  Outputs=3
  Digital Clock1 : DigitalClock  SampleTime=0.1
  From1 : From  Commented=on  GotoTag=MagRaw  TagVisibility=global
  Gain2 : Gain  Gain=1/280  OutDataTypeStr=double
  Low Pass Filter : Subsystem
  Mag data : Scope  Commented=on
      settings: ShowLegends=on  TimeRange=100  YMin=-15  YMax=50  SaveName=MagData
  Mux : Mux  Inputs=2
  Mux1 : Mux  Commented=on  Inputs=3
  Mux2 : Mux  Inputs=3
  Mux3 : Mux  Inputs=3
  Mux4 : Mux  Inputs=3
  Selector : Selector  InputPortWidth=2  Indices=[1]
  Selector1 : Selector  InputPortWidth=3  Indices=[1 2 3]
  Sine Wave : Sin  Commented=on  SineType=Sample based  Amplitude=6  Bias=-1  Samples=1000  SampleTime=0.01
  Sum4 : Sum  Inputs=|++
  Sys_ID_Data : Scope  Commented=on  NumInputPorts=5
      settings: ShowLegends=on  YMin=-5~-5~-5~-5~-5  YMax=5~5~5~5~5  SaveName=Sys_ID_Data_Record
  Temp : Scope  Commented=on
      settings: ShowLegends=on  TimeRange=100  YMin=47.83  YMax=48.03  SaveName=TempMeasure
  Time : Display
  Tune value Test : Scope  Commented=on
      settings: YMin=0.25  SaveName=UltraSound_Measure2
  UltraSound_Height : Scope  Commented=on  NumInputPorts=2
      settings: ShowLegends=on  TimeRange=1  YMin=0~-2  YMax=140~2  SaveName=UltrasoundHeight
  wires:
  Sine Wave/1 -> Tune value Test/1
  Digital Clock1/1 -> Time/1
  From1/1 -> Demux/1
  Demux/1 -> Mux1/1  "mag_x"
  Demux/2 -> Mux1/2  "mag_y"
  Demux/3 -> Mux1/3  "mag_z"
  Mux1/1 -> Mag data/1
  Demux2/1 -> Mux3/1  "p"
  Demux2/2 -> Mux3/2  "q"
  Demux2/3 -> Mux3/3  "r"
  [PQR_rates] -> Demux2/1
  [Height] -> Selector/1
  Demux1/1 -> Mux2/1  "Accel_X"
  Demux1/2 -> Mux2/2  "Accel_Y"
  Mux2/1 -> Accel/1
  Demux1/3 -> Mux2/3  "Accel_Z"
  [Accel] -> Demux1/1
  Data Type Conversion3/1 -> Sum4/1
  Constant1/1 -> Sum4/2
  Sum4/1 -> Gain2/1
  Gain2/1 -> Temp/1
  [TempMeasure] -> Data Type Conversion3/1
  LandingSwitch/1 -> UltraSound_Height/2  "ToggleLanding"
  LandingRef/1 -> Mux/1, Sys_ID_Data/3  "refHeight"
  Mux/1 -> UltraSound_Height/1
  Selector/1 -> Mux/2  "Height(centimeters)"
  Demux3/1 -> Mux4/1  "p"
  Demux3/2 -> Mux4/2  "q"
  Demux3/3 -> Mux4/3  "r"
  [PQR_Ctrl] -> Low Pass Filter/1(GyroMeasure)
  Low Pass Filter/1(GyroFiltered) -> Demux3/1
  Mux4/1 -> Body rates post processed - pre-conroller-input/1, Sys_ID_Data/2  "post_ctrl_attitude_rate"
  Mux3/1 -> Sys_ID_Data/1, Body rates/1  "pre_attitude_rate"
  [EulerAng] -> Selector1/1
  Selector1/1 -> Sys_ID_Data/4  "RollPitch_EulerAngles"
  Attitude_Cmd/1 -> Sys_ID_Data/5  "DesiredAttitude"

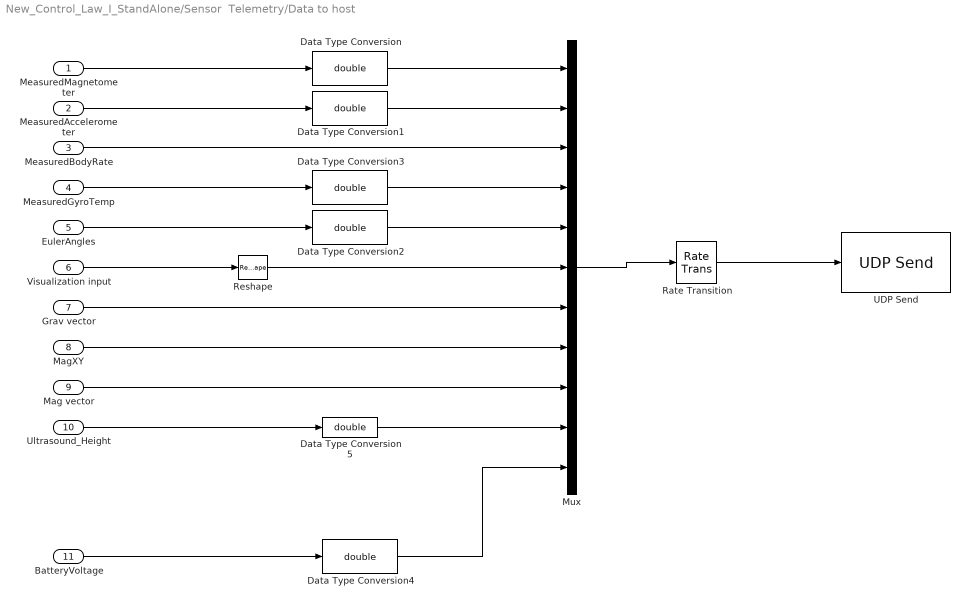
== system New_Control_Law_I_StandAlone/Sensor  Telemetry/Data to host ==
  MeasuredMagnetometer : Inport
  MeasuredAccelerometer : Inport  Port=2
  MeasuredBodyRate : Inport  Port=3
  MeasuredGyroTemp : Inport  Port=4
  EulerAngles : Inport  Port=5
  Visualization input : Inport  Port=6
  Grav vector : Inport  Port=7
  MagXY : Inport  Port=8
  Mag vector : Inport  Port=9
  Ultrasound_Height : Inport  Port=10
  BatteryVoltage : Inport  Port=11
  Data Type Conversion{,1..5} (6 alike) : DataTypeConversion  OutDataTypeStr=double
  Mux : Mux  Inputs=11
  Rate Transition : RateTransition  OutPortSampleTime=2/400
  Reshape : Reshape
  UDP Send : dspnetwork/UDP Send  remoteURL='192.168.1.2'  remotePort=25000  localURL='0.0.0.0'  localPortSource=Automatically determine  localPort=-1  sampletime=-1  blockPlatform=LINUX  separateLengthPort=0
  wires:
  MeasuredGyroTemp/1 -> Data Type Conversion3/1
  MeasuredAccelerometer/1 -> Data Type Conversion1/1
  MeasuredMagnetometer/1 -> Data Type Conversion/1
  EulerAngles/1 -> Data Type Conversion2/1
  MeasuredBodyRate/1 -> Mux/3
  Data Type Conversion3/1 -> Mux/4
  Data Type Conversion2/1 -> Mux/5
  Data Type Conversion1/1 -> Mux/2
  Data Type Conversion/1 -> Mux/1
  Mux/1 -> Rate Transition/1
  Rate Transition/1 -> UDP Send/1
  Visualization input/1 -> Reshape/1
  Reshape/1 -> Mux/6
  Grav vector/1 -> Mux/7
  MagXY/1 -> Mux/8
  Mag vector/1 -> Mux/9
  BatteryVoltage/1 -> Data Type Conversion4/1
  Data Type Conversion4/1 -> Mux/11
  Ultrasound_Height/1 -> Data Type Conversion5/1
  Data Type Conversion5/1 -> Mux/10

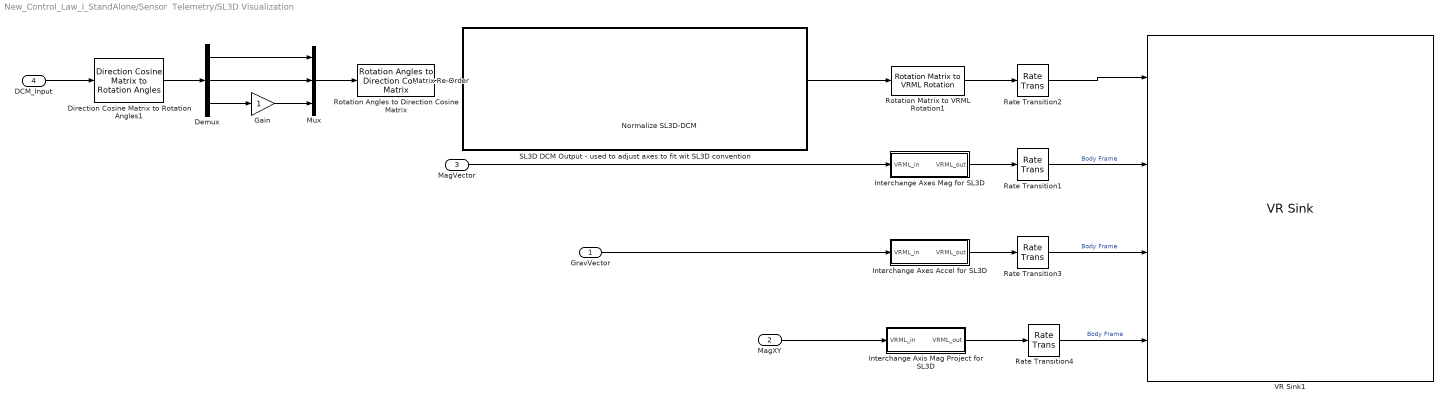
== system New_Control_Law_I_StandAlone/Sensor  Telemetry/SL3D Visualization ==
  GravVector : Inport
  MagXY : Inport  Port=2
  MagVector : Inport  Port=3
  DCM_Input : Inport  Port=4
  Demux : Demux  Outputs=3
  Direction Cosine Matrix to Rotation Angles1 : aerolibtransform2/Direction Cosine Matrix to Rotation Angles  rotationOrder=XYZ  lim=ZeroR3
      settings: AttributesFormatString=Rotation Order: %<rotationOrder>
  Gain : Gain  OutDataTypeStr=Inherit: Same as input
  "Interchange Axes Accel for SL3D " : Subsystem
  "Interchange Axes Mag for SL3D " : Subsystem
  Interchange Axis Mag Project for SL3D : Subsystem
  Matrix Re-Order : MATLAB Function  TreatAsAtomicUnit=on
  Mux : Mux  Inputs=3
  Normalize SL3D-DCM : Subsystem  TreatAsAtomicUnit=on
  Rate Transition{1..4} (4 alike) : RateTransition
  Rotation Angles to Direction Cosine Matrix : aerolibtransform2/Rotation Angles to Direction Cosine Matrix  rotationOrder=XYZ
  Rotation Matrix to VRML Rotation1 : vrlib/Utilities/Rotation Matrix to VRML Rotation  maxzero=1e-12
  SL3D DCM Output - used to adjust axes to fit wit SL3D convention : Subsystem
  VR Sink1 : vrlib/VR Sink  InstantiateOnLoad=on  SampleTime=0.02  ViewEnable=on  RemoteChange=off  RemoteView=off  FieldsWritten=Plane.rotation.4.1.1.double#mag_point.translation.3.1.1.double#grav_point.translation.3.1.1.double#mag_projection_point.translation.3.1.1.double  WorldFileName=vrml8_grav_2.WRL  AutoView=off  VideoDimensions=[]  AllowVariableSize=off
  wires:
  MagXY/1 -> Interchange Axis Mag Project for SL3D/1(VRML_in)
  Rate Transition2/1 -> VR Sink1/1
  Rate Transition1/1 -> VR Sink1/2  "Body Frame"
  Rate Transition3/1 -> VR Sink1/3  "Body Frame"
  Rate Transition4/1 -> VR Sink1/4  "Body Frame"
  Interchange Axis Mag Project for SL3D/1(VRML_out) -> Rate Transition4/1
  Rotation Angles to Direction Cosine Matrix/1 -> Matrix Re-Order/1(M_in)
  MagVector/1 -> "Interchange Axes Mag for SL3D "/1(VRML_in)
  "Interchange Axes Mag for SL3D "/1(VRML_out) -> Rate Transition1/1
  Mux/1 -> Rotation Angles to Direction Cosine Matrix/1
  Gain/1 -> Mux/3
  Demux/3 -> Gain/1
  Demux/2 -> Mux/2
  Demux/1 -> Mux/1
  Direction Cosine Matrix to Rotation Angles1/1 -> Demux/1
  Normalize SL3D-DCM/1(DCM_normalized) -> Rotation Matrix to VRML Rotation1/1
  Matrix Re-Order/1(M_out) -> Normalize SL3D-DCM/1(DCM)
  GravVector/1 -> "Interchange Axes Accel for SL3D "/1(VRML_in)
  DCM_Input/1 -> Direction Cosine Matrix to Rotation Angles1/1
  "Interchange Axes Accel for SL3D "/1(VRML_out) -> Rate Transition3/1
  Rotation Matrix to VRML Rotation1/1 -> Rate Transition2/1

== system New_Control_Law_I_StandAlone/Flight Controller/Supervisory Flight Controller/Attitude_Control/Offset ==
  AngleIn : Inport
  Demux : Demux  Outputs=2
  Demux3 : Demux  Outputs=2
  Examine Offset At Rest : Display
  Mux1 : Mux  Inputs=2
  Offset Constants : Constant  Value=[-0.6 +0.4]*0  OutDataTypeStr=single
  Sum : Sum  Inputs=|++
  Sum1 : Sum  Inputs=|++
  AngleOut : Outport
  wires:
  Mux1/1 -> AngleOut/1
  Sum/1 -> Mux1/1
  Sum1/1 -> Mux1/2
  Demux/2 -> Sum1/1
  AngleIn/1 -> Examine Offset At Rest/1, Demux/1
  Demux3/2 -> Sum1/2
  Demux3/1 -> Sum/2
  Demux/1 -> Sum/1
  Offset Constants/1 -> Demux3/1

== system New_Control_Law_I_StandAlone/Flight Controller/Supervisory Flight Controller/Attitude_Control/Roll Pitch Controller ==
  note: 250 to -250
  note: Stable Control
  errors : Inport
  Omega : Inport  Port=2
  MotorArmed : Inport  Port=3
  KP_OuterLoop_GAIN : Inport  Port=4
  KI_OuterLoop_GAIN : Inport  Port=5
  KP_InnerLoop_GAIN : Inport  Port=6
  K_PreGain_InnerLoop_GAIN : Inport  Port=7
  Attitude Command : Scope
      settings: SaveName=AttitudeRateCtrl_Cmd
  Data Type Conversion : DataTypeConversion  OutDataTypeStr=int16  RndMeth=Nearest
  Gain4 : Gain  Gain="[1.3 1.3]*4  %used to be *7"
  Ground : Ground
  Low Pass Filter : Subsystem
  Outer Loop Euler Angle Control Loop : Subsystem
  Saturation : Saturate  UpperLimit=250  LowerLimit=-250  OutDataTypeStr=int16
      settings: AttributesFormatString=%<LowerLimit>\nto\n%<UpperLimit>
  Sum : Sum  Inputs=|+-
  Terminator{,1..3} (4 alike) : Terminator
  Control_U : Outport
  Saturation Flag : Outport  Port=2
  wires:
  Saturation/1 -> Control_U/1
  Data Type Conversion/1 -> Saturation/1
  Outer Loop Euler Angle Control Loop/1(AttitudeRateCmd) -> Data Type Conversion/1  "PropSpeedCmd"
  MotorArmed/1 -> Outer Loop Euler Angle Control Loop/2(Motor Armed)
  Ground/1 -> Saturation Flag/1
  Omega/1 -> Low Pass Filter/1(GyroMeasure)
  errors/1 -> Gain4/1  "errors"
  Sum/1 -> Attitude Command/1, Outer Loop Euler Angle Control Loop/1(Attitude_Rate)
  Gain4/1 -> Sum/1
  Low Pass Filter/1(GyroFiltered) -> Sum/2
  KP_InnerLoop_GAIN/1 -> Terminator/1
  KP_OuterLoop_GAIN/1 -> Terminator1/1
  KI_OuterLoop_GAIN/1 -> Terminator2/1
  K_PreGain_InnerLoop_GAIN/1 -> Terminator3/1

== system New_Control_Law_I_StandAlone/Flight Controller/Supervisory Flight Controller/Attitude_Control/Yaw Counter-Active Control ==
  note: This Yaw Controller will prevent the drone from
      | rotating but does not tell the drone to rotate to a specified angle
  Euler_Yaw_Deg : Inport
  Rate_Gyro_R_deg : Inport  Port=2
  "Desired_yaw " : Inport  Port=3
  Add1 : Sum  Inputs=+-  AccumDataTypeStr=single  OutDataTypeStr=single
  Add2 : Sum  Inputs=+-  AccumDataTypeStr=single  OutDataTypeStr=single
  Data Type Conversion : DataTypeConversion  OutDataTypeStr=int16
  Discrete Derivative : simulink/Discrete/Discrete Derivative  gainval=1.0  ICPrevScaledInput=0.0  InputProcessing=Inherited  OutMin=[]  OutMax=[]  OutDataType=fixdt(1, 16)  OutScaling=2^-10  DoSatur=off
  InterChange_Axis : Gain  Gain=-1  ParamDataTypeStr=single  OutDataTypeStr=single
      settings: AttributesFormatString=%<Gain>
  To Degrees2 : Gain  Gain=180/pi  ParamDataTypeStr=single  OutDataTypeStr=single
      settings: AttributesFormatString=%<Gain>
  To Degrees3 : Gain  ParamDataTypeStr=single  OutDataTypeStr=single
      settings: AttributesFormatString=%<Gain>
  Yaw_contribution : Gain  Gain=2.5*2  ParamDataTypeStr=single  OutDataTypeStr=single
      settings: AttributesFormatString=%<Gain>
  Yaw_contribution1 : Gain  Gain=0.06  ParamDataTypeStr=single  OutDataTypeStr=single
      settings: AttributesFormatString=%<Gain>
  YawCommand : Outport
  wires:
  Yaw_contribution1/1 -> Data Type Conversion/1
  To Degrees3/1 -> Add1/2
  Euler_Yaw_Deg/1 -> InterChange_Axis/1
  Add1/1 -> Yaw_contribution1/1
  Yaw_contribution/1 -> Add1/1
  Add2/1 -> Yaw_contribution/1
  InterChange_Axis/1 -> Discrete Derivative/1
  Discrete Derivative/1 -> Add2/1
  To Degrees2/1 -> Add2/2
  "Desired_yaw "/1 -> To Degrees2/1
  Rate_Gyro_R_deg/1 -> To Degrees3/1
  Data Type Conversion/1 -> YawCommand/1

== system New_Control_Law_I_StandAlone/Flight Controller/Supervisory Flight Controller/Attitude_Control/Yaw Signal Builder  ==
  Demux : Demux  Tag=STV Demux  Outputs=1
  FromWs : FromWorkspace  Tag=STV FromWs  VariableName=tuvar
      SigBuilderData=|
      | common.afterFinalStr = 'Extrapolate'
      | common.sampleTime = '-1'
      | dataSet.timeRange = [0 20]
      | dataSet.name = 'Group 1'
      | sbobj.Groups.Name = 'Group 1'
      | sbobj.Groups.Signals.Name = 'Signal 1'
      | sbobj.Groups.Signals.XData = [0 10 10 12.5 12.5 15 15 20]
      | sbobj.Groups.Signals.YData = [0 0 2 2 -2 -2 0 0]
      | sbobj.Groups.TimeRange = [0 20]
  Signal 1 : Outport  Tag=STV Outport
  wires:
  Demux/1 -> Signal 1/1
  FromWs/1 -> Demux/1

== system New_Control_Law_I_StandAlone/Navigation/CheckSum Pre-Processing/Accelerometer Processing ==
  Raw Data : Inport
  CheckSum Flag : Inport  Port=2
  Holding Value : Inport  Port=3
  Calculate Accel Data : Subsystem  Commented=through
  CheckSum Correction : Subsystem
  Processed Data : Outport
  wires:
  Holding Value/1 -> CheckSum Correction/3(Holding Value)
  Calculate Accel Data/1(Processed Accel Data) -> CheckSum Correction/1(CalculatedData)
  CheckSum Correction/1(Pre-Processed Height) -> Processed Data/1
  Raw Data/1 -> Calculate Accel Data/1(Raw Accel Data)
  CheckSum Flag/1 -> CheckSum Correction/2(CheckSumFlag)

== system New_Control_Law_I_StandAlone/Navigation/CheckSum Pre-Processing/Magnetometer ==
  Magnetometer : Inport
  CheckSum Flag : Inport  Port=2
  Holding Value : Inport  Port=3
  CheckSum Correction : Subsystem
  Process Raw Mag Data : Subsystem  Commented=through
  Processed Data : Outport
  wires:
  Holding Value/1 -> CheckSum Correction/3(Holding Value)
  Process Raw Mag Data/1(ProcessedData) -> CheckSum Correction/1(CalculatedData)
  Magnetometer/1 -> Process Raw Mag Data/1(Magnetometer)
  CheckSum Correction/1(Pre-Processed Data) -> Processed Data/1
  CheckSum Flag/1 -> CheckSum Correction/2(CheckSumFlag)

== system New_Control_Law_I_StandAlone/Navigation/CheckSum Pre-Processing/RateGyro Processing ==
  Raw Data : Inport
  CheckSum Flag : Inport  Port=2
  Holding Value : Inport  Port=3
  CheckSum Correction : Subsystem
  Process Data : Subsystem  Commented=through
  Processed Data : Outport
  wires:
  Holding Value/1 -> CheckSum Correction/3(Holding Value)
  Process Data/1(Processed Data) -> CheckSum Correction/1(CalculatedData)
  Raw Data/1 -> Process Data/1(Raw Data)
  CheckSum Correction/1(Pre-Processed Height) -> Processed Data/1
  CheckSum Flag/1 -> CheckSum Correction/2(CheckSumFlag)
